simulink model "AFC_FFNN_trainlm_15_15_15_15_Apr_1_2020_M"  (R2021b)
settings: Solver=ode15s  StartTime=0.0  StopTime=30  MaxStep=0.01  RelTol=1e-3
libraries: neural x66
(part 3 of 3)

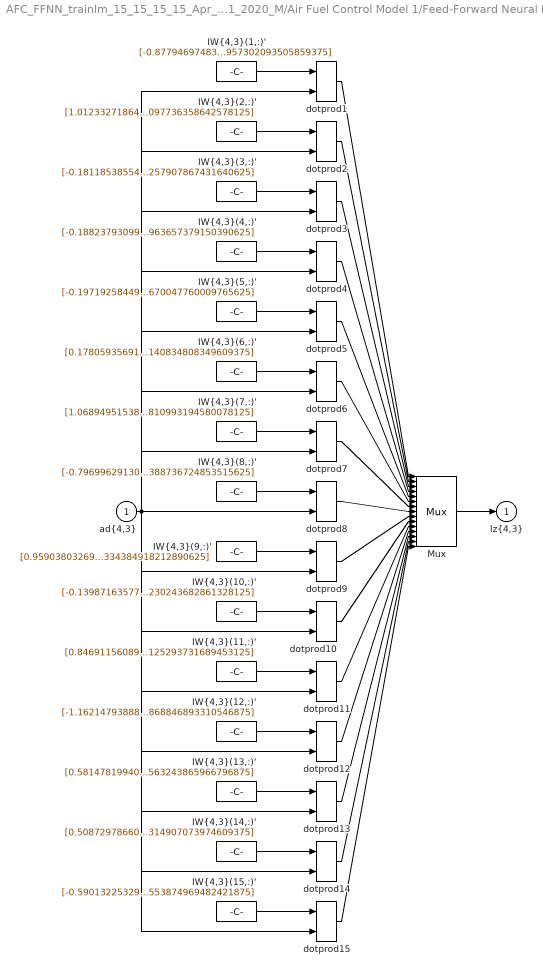
== system AFC_FFNN_trainlm_15_15_15_15_Apr_1_2020_M/Air Fuel Control Model 1/Feed-Forward Neural Network/Layer 4/LW{4,3} ==
  "ad{4,3}" : Inport  PortDimensions=15
      mask Display: e = 0.06;c1 = [120 230 180]/255;c2 = ([120 230 180]+0)/(256+128);c3 = ([120 230 180]+128)/(256+128);patch([0 1 1 0],[0 0 1 1],c1);patch([0 1 1 1-e 1-e 0+e],[0 0 1 1-e 0+e 0+e],c2);patch([0 0 1 1-e 0+e 0+e],[0 1 1 1-e 1-e 0+e],c3);plot([0 1 1 0 0],[0 0 1 1 0]);
  "IW{4,3}(1,:)'" : Constant  Value=[-0.87794697483855188568924177161534316837787628173828125;0.78511271343722122129094032061402685940265655517578125;0.50154215742376317965778298457735218107700347900390625;0.2817626613878057018069966943585313856601715087890625;-0.0447481608464237456956880123470909893512725830078125;-0.627329734092003210577104255207814276218414306640625;0.55694927688418560673966339891194365918636322021484375;-0.7464244490308360457930803022463805973529815673828125;0.54695272101903003036937889191904105246067047119140625;-0.30506713981724431494768623451818712055683135986328125;0.1330716598486472446172257377838832326233386993408203125;-0.36209291832798218280231594690121710300445556640625;0.1493922263287312812707341436180286109447479248046875;0.721901657154491172008192734210751950740814208984375;0.57616554688412902063276987973949871957302093505859375]
      mask Display: e = 0.06;c1 = [120 150 230]/255;c2 = ([120 150 230]+0)/383;c3 = ([120 150 230]+128)/383;patch([0 1 1 0],[0 0 1 1],c1);patch([0 1 1 1-e 1-e 0+e],[0 0 1 1-e 0+e 0+e],c2);patch([0 0 1 1-e 0+e 0+e],[0 1 1 1-e 1-e 0+e],c3);plot([0 1 1 0 0],[0 0 1 1 0]);disp('weights');
  "IW{4,3}(10,:)'" : Constant  Value=[-0.1398716357765525108991511160638765431940555572509765625;0.082048350523899193920129846446798183023929595947265625;0.0035940872365181979718185001360097885481081902980804443359375;0.61364753046270592573563362748245708644390106201171875;-0.1449570401924471507726366326096467673778533935546875;-0.621340313949121370029615718522109091281890869140625;-0.63152240904524414855103486843290738761425018310546875;0.18129030978633087212159580303705297410488128662109375;0.70918842566612350086785454550408758223056793212890625;0.444294267001949183537590215564705431461334228515625;0.3511170382244828136464320778031833469867706298828125;0.9678951234339694398300935063161887228488922119140625;-0.43500142397416130535248157684691250324249267578125;-0.292582299598873607493487725150771439075469970703125;-0.72720331825824502391952819380094297230243682861328125]
      mask Display: e = 0.06;c1 = [120 150 230]/255;c2 = ([120 150 230]+0)/383;c3 = ([120 150 230]+128)/383;patch([0 1 1 0],[0 0 1 1],c1);patch([0 1 1 1-e 1-e 0+e],[0 0 1 1-e 0+e 0+e],c2);patch([0 0 1 1-e 0+e 0+e],[0 1 1 1-e 1-e 0+e],c3);plot([0 1 1 0 0],[0 0 1 1 0]);disp('weights');
  "IW{4,3}(11,:)'" : Constant  Value=[0.8469115608906976344627537400810979306697845458984375;-0.311598694041631762985389286768622696399688720703125;-0.4555113193085655876046757839503698050975799560546875;0.2257560371225231232727992392028681933879852294921875;-0.1536297879854113812569949004682712256908416748046875;0.6246753040878669782642873542499728500843048095703125;-0.618342893403056592660504975356161594390869140625;0.87203667944872542694412231867318041622638702392578125;0.312036102352537036974666762034757994115352630615234375;0.53507958236281094599462448968552052974700927734375;1.0606246666988126126085489886463619768619537353515625;0.459631876268668915219706150310230441391468048095703125;0.87284799201372553767441786476410925388336181640625;0.3642501475629236207254280088818632066249847412109375;0.32478448388082625797323998995125293731689453125]
      mask Display: e = 0.06;c1 = [120 150 230]/255;c2 = ([120 150 230]+0)/383;c3 = ([120 150 230]+128)/383;patch([0 1 1 0],[0 0 1 1],c1);patch([0 1 1 1-e 1-e 0+e],[0 0 1 1-e 0+e 0+e],c2);patch([0 0 1 1-e 0+e 0+e],[0 1 1 1-e 1-e 0+e],c3);plot([0 1 1 0 0],[0 0 1 1 0]);disp('weights');
  "IW{4,3}(12,:)'" : Constant  Value=[-1.1621479388899036422344579477794468402862548828125;-0.88605701259143276882213058343040756881237030029296875;0.66235299370133871033061723210266791284084320068359375;-0.07077567879171035858387739381214487366378307342529296875;-0.27211799036489470182687000487931072711944580078125;0.72261696466571867514261384712881408631801605224609375;0.55103460441041873796308436794788576662540435791015625;0.183429125512546919996026417720713652670383453369140625;-0.344389971699303687469040369251160882413387298583984375;-0.91398906043296601620085084505262784659862518310546875;0.57553134575504871772722026435076259076595306396484375;-0.5461197652611726738314246176742017269134521484375;-0.708172309786351039662122275331057608127593994140625;0.3874597979113507673076810533530078828334808349609375;-0.9807440176240997953271971709909848868846893310546875]
      mask Display: e = 0.06;c1 = [120 150 230]/255;c2 = ([120 150 230]+0)/383;c3 = ([120 150 230]+128)/383;patch([0 1 1 0],[0 0 1 1],c1);patch([0 1 1 1-e 1-e 0+e],[0 0 1 1-e 0+e 0+e],c2);patch([0 0 1 1-e 0+e 0+e],[0 1 1 1-e 1-e 0+e],c3);plot([0 1 1 0 0],[0 0 1 1 0]);disp('weights');
  "IW{4,3}(13,:)'" : Constant  Value=[0.58147819940035194719030187116004526615142822265625;0.66671058191855803176650852037710137665271759033203125;0.82713190563479377370725842411047779023647308349609375;-0.7444983522659407437771506010903976857662200927734375;0.40638725377066275967763431253843009471893310546875;0.6613316222049554493622736117686145007610321044921875;0.80557784201437854232352719918708316981792449951171875;0.18716756979224313806042800933937542140483856201171875;0.65199814324099103490794959725462831556797027587890625;-0.851432769005782130733450685511343181133270263671875;-0.283226375762959836634991006576456129550933837890625;0.63658715279129207686992231174372136592864990234375;-0.4675533643194753619098946728627197444438934326171875;-0.3662417914291811182891933640348725020885467529296875;0.5858475047353255416027195678907446563243865966796875]
      mask Display: e = 0.06;c1 = [120 150 230]/255;c2 = ([120 150 230]+0)/383;c3 = ([120 150 230]+128)/383;patch([0 1 1 0],[0 0 1 1],c1);patch([0 1 1 1-e 1-e 0+e],[0 0 1 1-e 0+e 0+e],c2);patch([0 0 1 1-e 0+e 0+e],[0 1 1 1-e 1-e 0+e],c3);plot([0 1 1 0 0],[0 0 1 1 0]);disp('weights');
  "IW{4,3}(14,:)'" : Constant  Value=[0.5087297866062605589121403681929223239421844482421875;0.188991786837609809790450299260555766522884368896484375;0.62040033157972629407339582030544988811016082763671875;-1.3169260075057744874271747903549112379550933837890625;-0.29726006120487280526276663294993340969085693359375;0.58833087830961405817475906587787903845310211181640625;-0.647600995689554093104334242525510489940643310546875;-0.24550691338193553203694818876101635396480560302734375;-0.06475428417855148832682488091450068168342113494873046875;-0.8097839625485210302002769822138361632823944091796875;-0.69917278753788469902730184912797994911670684814453125;1.0912869846500914405851290212012827396392822265625;-0.5144129881700150175305452648899517953395843505859375;0.79022942493543701925062805457855574786663055419921875;2.26916884611590941034364732331596314907073974609375]
      mask Display: e = 0.06;c1 = [120 150 230]/255;c2 = ([120 150 230]+0)/383;c3 = ([120 150 230]+128)/383;patch([0 1 1 0],[0 0 1 1],c1);patch([0 1 1 1-e 1-e 0+e],[0 0 1 1-e 0+e 0+e],c2);patch([0 0 1 1-e 0+e 0+e],[0 1 1 1-e 1-e 0+e],c3);plot([0 1 1 0 0],[0 0 1 1 0]);disp('weights');
  "IW{4,3}(15,:)'" : Constant  Value=[-0.59013225329123086826399458004743792116641998291015625;0.68362536896318470969191594122094102203845977783203125;0.51268345737815590457131520452094264328479766845703125;0.73534210419389067769913026495487429201602935791015625;-0.722623441227063789682460992480628192424774169921875;0.4950531857779767452854002840467728674411773681640625;0.0039842636764119976344744600282865576446056365966796875;0.58761554450892272694062512528034858405590057373046875;-0.58080760878334014574164712030324153602123260498046875;-0.32518728515714634408340089066768996417522430419921875;0.8049732768928656856388670348678715527057647705078125;-0.34826732744436983413294228739687241613864898681640625;0.7186328066455740515294792203349061310291290283203125;-0.3212892271896301554789943111245520412921905517578125;0.334461971693696902274695048618013970553874969482421875]
      mask Display: e = 0.06;c1 = [120 150 230]/255;c2 = ([120 150 230]+0)/383;c3 = ([120 150 230]+128)/383;patch([0 1 1 0],[0 0 1 1],c1);patch([0 1 1 1-e 1-e 0+e],[0 0 1 1-e 0+e 0+e],c2);patch([0 0 1 1-e 0+e 0+e],[0 1 1 1-e 1-e 0+e],c3);plot([0 1 1 0 0],[0 0 1 1 0]);disp('weights');
  "IW{4,3}(2,:)'" : Constant  Value=[1.0123327186491437590376563093741424381732940673828125;1.098571239363774765251946519128978252410888671875;1.0135981388833539273974793104571290314197540283203125;0.190480505210553541228790663808467797935009002685546875;-0.61174606671621578612985103973187506198883056640625;0.001871022357728312213165366983957937918603420257568359375;-0.77443426081876098887590842423378489911556243896484375;0.8933686526028079555317162885330617427825927734375;-0.05576797680758034669867839738799375481903553009033203125;0.337953956266565713750793520375736989080905914306640625;-0.1422828298717915551652168915097718127071857452392578125;0.7575526069568947473698017347487621009349822998046875;-0.4194139141820738547750124780577607452869415283203125;0.66597243693851115864390521892346441745758056640625;-0.83251762673654561286440412004594691097736358642578125]
      mask Display: e = 0.06;c1 = [120 150 230]/255;c2 = ([120 150 230]+0)/383;c3 = ([120 150 230]+128)/383;patch([0 1 1 0],[0 0 1 1],c1);patch([0 1 1 1-e 1-e 0+e],[0 0 1 1-e 0+e 0+e],c2);patch([0 0 1 1-e 0+e 0+e],[0 1 1 1-e 1-e 0+e],c3);plot([0 1 1 0 0],[0 0 1 1 0]);disp('weights');
  "IW{4,3}(3,:)'" : Constant  Value=[-0.1811853855497163878762734157135128043591976165771484375;-0.5960881500003465394144086531014181673526763916015625;0.441979396271819202635100509723997674882411956787109375;0.7947734403244870460270021794713102281093597412109375;-0.1868516521181187162170544979744590818881988525390625;-1.0137783650240865807035106627154164016246795654296875;0.33786822212746570048835792476893402636051177978515625;0.40355475766253279257256281198351643979549407958984375;0.420947115571197294503491548312013037502765655517578125;-0.926163186954993111754674828262068331241607666015625;0.223759547769176114773159724791184999048709869384765625;0.8695239017841422946020202289219014346599578857421875;-0.4197462449481268453865823175874538719654083251953125;0.8011093081199256449309586969320662319660186767578125;0.018384635967900353481496722451993264257907867431640625]
      mask Display: e = 0.06;c1 = [120 150 230]/255;c2 = ([120 150 230]+0)/383;c3 = ([120 150 230]+128)/383;patch([0 1 1 0],[0 0 1 1],c1);patch([0 1 1 1-e 1-e 0+e],[0 0 1 1-e 0+e 0+e],c2);patch([0 0 1 1-e 0+e 0+e],[0 1 1 1-e 1-e 0+e],c3);plot([0 1 1 0 0],[0 0 1 1 0]);disp('weights');
  "IW{4,3}(4,:)'" : Constant  Value=[-0.1882379309967188996122189337256713770329952239990234375;0.89920767196481643512839809773140586912631988525390625;-0.7963876016425033288470558545668609440326690673828125;-0.00942815664871557955473146961367092444561421871185302734375;0.829359092604627701206254641874693334102630615234375;0.386189766269589729308364667303976602852344512939453125;0.56148647590458555800552176151541061699390411376953125;-0.7148532027965293078608510768390260636806488037109375;0.206937721753990666595512948333634994924068450927734375;0.265127551825350249448121076056850142776966094970703125;-0.288570537994503606427088016062043607234954833984375;0.55649333418204793844097366672940552234649658203125;-0.8044316294032711756045728179742582142353057861328125;0.5612939377825572062619130520033650100231170654296875;0.73878778787138055239580580746405757963657379150390625]
      mask Display: e = 0.06;c1 = [120 150 230]/255;c2 = ([120 150 230]+0)/383;c3 = ([120 150 230]+128)/383;patch([0 1 1 0],[0 0 1 1],c1);patch([0 1 1 1-e 1-e 0+e],[0 0 1 1-e 0+e 0+e],c2);patch([0 0 1 1-e 0+e 0+e],[0 1 1 1-e 1-e 0+e],c3);plot([0 1 1 0 0],[0 0 1 1 0]);disp('weights');
  "IW{4,3}(5,:)'" : Constant  Value=[-0.197192584497892564598942044540308415889739990234375;-0.5186706284037716496726488912827335298061370849609375;0.510598952565356256627637776546180248260498046875;-0.5671754650160829580585186704411171376705169677734375;0.6290541607610642405035150659386999905109405517578125;-0.593972205237285333367935891146771609783172607421875;0.56367557776157273252692903042770922183990478515625;-0.2391886933281599514344861745485104620456695556640625;0.2483531137671775024244880114565603435039520263671875;-0.4021721998758012173169618108659051358699798583984375;-0.8607509458168005611611306449049152433872222900390625;-0.6985358795817571131436807263526134192943572998046875;0.09485220801825988701239111833274364471435546875;-0.42931368309029682706068342668004333972930908203125;0.1919537785317848577193444725708104670047760009765625]
      mask Display: e = 0.06;c1 = [120 150 230]/255;c2 = ([120 150 230]+0)/383;c3 = ([120 150 230]+128)/383;patch([0 1 1 0],[0 0 1 1],c1);patch([0 1 1 1-e 1-e 0+e],[0 0 1 1-e 0+e 0+e],c2);patch([0 0 1 1-e 0+e 0+e],[0 1 1 1-e 1-e 0+e],c3);plot([0 1 1 0 0],[0 0 1 1 0]);disp('weights');
  "IW{4,3}(6,:)'" : Constant  Value=[0.1780593569155609345866508874678402207791805267333984375;0.51295577667334602001147914052125997841358184814453125;-0.2488674401089323584557178037357516586780548095703125;-0.52678522851250020320179601185373030602931976318359375;0.2838564984986617911744133380125276744365692138671875;0.7661743777528631227369260159321129322052001953125;-0.395950144348631460911036583638633601367473602294921875;0.66942143988391222819700487889349460601806640625;-0.70887282503045512260797522685606963932514190673828125;0.420234137501336479925129196999478153884410858154296875;-0.3134912186981633208660014133783988654613494873046875;-0.31435256189060167830717773540527559816837310791015625;0.244775657654162426268840135890059173107147216796875;0.55164477009675305652081078733317553997039794921875;-0.332656944910989016417346419984824024140834808349609375]
      mask Display: e = 0.06;c1 = [120 150 230]/255;c2 = ([120 150 230]+0)/383;c3 = ([120 150 230]+128)/383;patch([0 1 1 0],[0 0 1 1],c1);patch([0 1 1 1-e 1-e 0+e],[0 0 1 1-e 0+e 0+e],c2);patch([0 0 1 1-e 0+e 0+e],[0 1 1 1-e 1-e 0+e],c3);plot([0 1 1 0 0],[0 0 1 1 0]);disp('weights');
  "IW{4,3}(7,:)'" : Constant  Value=[1.0689495153859998044509893588838167488574981689453125;-0.48233115858616770754707658852566964924335479736328125;0.0623997962497397640202478896753746084868907928466796875;0.7931784702682118659566867790999822318553924560546875;-0.1412504172778643596330994114396162331104278564453125;0.354917548973855356830853224892052821815013885498046875;0.82917133329300707345055343466810882091522216796875;-0.01606084327905706043981837183309835381805896759033203125;-0.50281957762533469047383505312609486281871795654296875;-0.55237366074994465048320080313715152442455291748046875;-0.69503012315862633396790215556393377482891082763671875;0.5879995412831016121657512485398910939693450927734375;0.2442786986054261699763401338714174926280975341796875;-0.906706083575766541571283596567809581756591796875;-0.79723882076575158794895514802192337810993194580078125]
      mask Display: e = 0.06;c1 = [120 150 230]/255;c2 = ([120 150 230]+0)/383;c3 = ([120 150 230]+128)/383;patch([0 1 1 0],[0 0 1 1],c1);patch([0 1 1 1-e 1-e 0+e],[0 0 1 1-e 0+e 0+e],c2);patch([0 0 1 1-e 0+e 0+e],[0 1 1 1-e 1-e 0+e],c3);plot([0 1 1 0 0],[0 0 1 1 0]);disp('weights');
  "IW{4,3}(8,:)'" : Constant  Value=[-0.79699629130861981973765750808524899184703826904296875;0.81516845271742022216443501747562550008296966552734375;-0.10325580243793168466748255696074920706450939178466796875;-0.12629156005249997374306758501916192471981048583984375;0.001780542089853565101975618745200335979461669921875;-0.626000500890068867221316395443864166736602783203125;0.022190916577181425684006654819313553161919116973876953125;-0.161612416675443737457129600443295203149318695068359375;-0.278241324625298769301906531836721114814281463623046875;-0.5271108348563908752026918591582216322422027587890625;1.044387681269747236711964433197863399982452392578125;0.6362087423169793254373871604911983013153076171875;-0.3089480363396763795691413179156370460987091064453125;0.209791869896167992859403739203116856515407562255859375;1.9123701938083981222149532186449505388736724853515625]
      mask Display: e = 0.06;c1 = [120 150 230]/255;c2 = ([120 150 230]+0)/383;c3 = ([120 150 230]+128)/383;patch([0 1 1 0],[0 0 1 1],c1);patch([0 1 1 1-e 1-e 0+e],[0 0 1 1-e 0+e 0+e],c2);patch([0 0 1 1-e 0+e 0+e],[0 1 1 1-e 1-e 0+e],c3);plot([0 1 1 0 0],[0 0 1 1 0]);disp('weights');
  "IW{4,3}(9,:)'" : Constant  Value=[0.95903803269837906153583162449649535119533538818359375;0.1797639268302933801546572567531256936490535736083984375;0.47397786629673699376752438183757476508617401123046875;0.84812206479178875451196972790057770907878875732421875;-0.6216250145664379278542810425278730690479278564453125;1.0559711154374264996391730164759792387485504150390625;1.003550640057164766716368831112049520015716552734375;-0.16921524677973753814086421698448248207569122314453125;-0.388523293891599064142639008423429913818836212158203125;0.64295138099676096832268967773416079580783843994140625;-0.7218467335780027749336795750423334538936614990234375;0.755669871799011350077535098535008728504180908203125;-0.7771348063268403993930633077980019152164459228515625;-0.9635683972860367152435401294496841728687286376953125;0.0846822230062286573915031340220593847334384918212890625]
      mask Display: e = 0.06;c1 = [120 150 230]/255;c2 = ([120 150 230]+0)/383;c3 = ([120 150 230]+128)/383;patch([0 1 1 0],[0 0 1 1],c1);patch([0 1 1 1-e 1-e 0+e],[0 0 1 1-e 0+e 0+e],c2);patch([0 0 1 1-e 0+e 0+e],[0 1 1 1-e 1-e 0+e],c3);plot([0 1 1 0 0],[0 0 1 1 0]);disp('weights');
  Mux : Mux  Inputs=15
      mask Display: e = 0.06;c1 = [120 150 230]/255;c2 = ([120 150 230]+0)/383;c3 = ([120 150 230]+128)/383;patch([0 1 1 0],[0 0 1 1],c1);patch([0 1 1 1-e 1-e 0+e],[0 0 1 1-e 0+e 0+e],c2);patch([0 0 1 1-e 0+e 0+e],[0 1 1 1-e 1-e 0+e],c3);plot([0 1 1 0 0],[0 0 1 1 0]);disp('Mux');
  dotprod{1..15} (15 alike) : neural/Weight Functions/dotprod
  "lz{4,3}" : Outport
      mask Display: e = 0.06;c1 = [120 230 180]/255;c2 = ([120 230 180]+0)/(256+128);c3 = ([120 230 180]+128)/(256+128);patch([0 1 1 0],[0 0 1 1],c1);patch([0 1 1 1-e 1-e 0+e],[0 0 1 1-e 0+e 0+e],c2);patch([0 0 1 1-e 0+e 0+e],[0 1 1 1-e 1-e 0+e],c3);plot([0 1 1 0 0],[0 0 1 1 0]);
  wires:
  "IW{4,3}(1,:)'"/1 -> dotprod1/1
  "ad{4,3}"/1 -> dotprod1/2, dotprod2/2, dotprod3/2, dotprod4/2, dotprod5/2, dotprod6/2, dotprod7/2, dotprod8/2, dotprod9/2, dotprod10/2, dotprod11/2, dotprod12/2, dotprod13/2, dotprod14/2, dotprod15/2
  dotprod1/1 -> Mux/1
  "IW{4,3}(2,:)'"/1 -> dotprod2/1
  dotprod2/1 -> Mux/2
  "IW{4,3}(3,:)'"/1 -> dotprod3/1
  dotprod3/1 -> Mux/3
  "IW{4,3}(4,:)'"/1 -> dotprod4/1
  dotprod4/1 -> Mux/4
  "IW{4,3}(5,:)'"/1 -> dotprod5/1
  dotprod5/1 -> Mux/5
  "IW{4,3}(6,:)'"/1 -> dotprod6/1
  dotprod6/1 -> Mux/6
  "IW{4,3}(7,:)'"/1 -> dotprod7/1
  dotprod7/1 -> Mux/7
  "IW{4,3}(8,:)'"/1 -> dotprod8/1
  dotprod8/1 -> Mux/8
  "IW{4,3}(9,:)'"/1 -> dotprod9/1
  dotprod9/1 -> Mux/9
  "IW{4,3}(10,:)'"/1 -> dotprod10/1
  dotprod10/1 -> Mux/10
  "IW{4,3}(11,:)'"/1 -> dotprod11/1
  dotprod11/1 -> Mux/11
  "IW{4,3}(12,:)'"/1 -> dotprod12/1
  dotprod12/1 -> Mux/12
  "IW{4,3}(13,:)'"/1 -> dotprod13/1
  dotprod13/1 -> Mux/13
  "IW{4,3}(14,:)'"/1 -> dotprod14/1
  dotprod14/1 -> Mux/14
  "IW{4,3}(15,:)'"/1 -> dotprod15/1
  dotprod15/1 -> Mux/15
  Mux/1 -> "lz{4,3}"/1

== system AFC_FFNN_trainlm_15_15_15_15_Apr_1_2020_M/Air Fuel Control Model 1/Feed-Forward Neural Network/Layer 5/Delays 1 ==
  "p{5}" : Inport  PortDimensions=15
      mask Display: e = 0.06;c1 = [120 230 180]/255;c2 = ([120 230 180]+0)/(256+128);c3 = ([120 230 180]+128)/(256+128);patch([0 1 1 0],[0 0 1 1],c1);patch([0 1 1 1-e 1-e 0+e],[0 0 1 1-e 0+e 0+e],c2);patch([0 0 1 1-e 0+e 0+e],[0 1 1 1-e 1-e 0+e],c3);plot([0 1 1 0 0],[0 0 1 1 0]);
  mux : Mux  Inputs=1
      mask Display: e = 0.06;c1 = [120 150 230]/255;c2 = ([120 150 230]+0)/383;c3 = ([120 150 230]+128)/383;patch([0 1 1 0],[0 0 1 1],c1);patch([0 1 1 1-e 1-e 0+e],[0 0 1 1-e 0+e 0+e],c2);patch([0 0 1 1-e 0+e 0+e],[0 1 1 1-e 1-e 0+e],c3);plot([0 1 1 0 0],[0 0 1 1 0]);disp('Mux')
  "pd{5,4}" : Outport
      mask Display: e = 0.06;c1 = [120 230 180]/255;c2 = ([120 230 180]+0)/(256+128);c3 = ([120 230 180]+128)/(256+128);patch([0 1 1 0],[0 0 1 1],c1);patch([0 1 1 1-e 1-e 0+e],[0 0 1 1-e 0+e 0+e],c2);patch([0 0 1 1-e 0+e 0+e],[0 1 1 1-e 1-e 0+e],c3);plot([0 1 1 0 0],[0 0 1 1 0]);
  wires:
  "p{5}"/1 -> mux/1
  mux/1 -> "pd{5,4}"/1

== system AFC_FFNN_trainlm_15_15_15_15_Apr_1_2020_M/Air Fuel Control Model 1/Feed-Forward Neural Network/Layer 5/LW{5,4} ==
  "ad{5,4}" : Inport  PortDimensions=15
      mask Display: e = 0.06;c1 = [120 230 180]/255;c2 = ([120 230 180]+0)/(256+128);c3 = ([120 230 180]+128)/(256+128);patch([0 1 1 0],[0 0 1 1],c1);patch([0 1 1 1-e 1-e 0+e],[0 0 1 1-e 0+e 0+e],c2);patch([0 0 1 1-e 0+e 0+e],[0 1 1 1-e 1-e 0+e],c3);plot([0 1 1 0 0],[0 0 1 1 0]);
  "IW{5,4}(1,:)'" : Constant  Value=[0.19989144575989870045162888345657847821712493896484375;0.52004998107383826333460774549166671931743621826171875;-0.752803453565191293961333940387703478336334228515625;0.428612666235617612020547539941617287695407867431640625;0.585595362040919109603009928832761943340301513671875;-0.3562629890878257210573565316735766828060150146484375;0.5961351434564565732188157198834232985973358154296875;-0.74671233793534808054204177096835337579250335693359375;0.311648142554934948211808887208462692797183990478515625;-0.66544677705073718154693551696254871785640716552734375;0.6726563067034001530686282421811483800411224365234375;-0.65963526623929624737030508185853250324726104736328125;-0.377066482508966682729578678845427930355072021484375;0.1906180581610984192675317672183155082166194915771484375;0.1745649841584534234240067007704055868089199066162109375]
      mask Display: e = 0.06;c1 = [120 150 230]/255;c2 = ([120 150 230]+0)/383;c3 = ([120 150 230]+128)/383;patch([0 1 1 0],[0 0 1 1],c1);patch([0 1 1 1-e 1-e 0+e],[0 0 1 1-e 0+e 0+e],c2);patch([0 0 1 1-e 0+e 0+e],[0 1 1 1-e 1-e 0+e],c3);plot([0 1 1 0 0],[0 0 1 1 0]);disp('weights');
  Mux : Mux  Inputs=1
      mask Display: e = 0.06;c1 = [120 150 230]/255;c2 = ([120 150 230]+0)/383;c3 = ([120 150 230]+128)/383;patch([0 1 1 0],[0 0 1 1],c1);patch([0 1 1 1-e 1-e 0+e],[0 0 1 1-e 0+e 0+e],c2);patch([0 0 1 1-e 0+e 0+e],[0 1 1 1-e 1-e 0+e],c3);plot([0 1 1 0 0],[0 0 1 1 0]);disp('Mux');
  dotprod1 : neural/Weight Functions/dotprod
  "lz{5,4}" : Outport
      mask Display: e = 0.06;c1 = [120 230 180]/255;c2 = ([120 230 180]+0)/(256+128);c3 = ([120 230 180]+128)/(256+128);patch([0 1 1 0],[0 0 1 1],c1);patch([0 1 1 1-e 1-e 0+e],[0 0 1 1-e 0+e 0+e],c2);patch([0 0 1 1-e 0+e 0+e],[0 1 1 1-e 1-e 0+e],c3);plot([0 1 1 0 0],[0 0 1 1 0]);
  wires:
  "IW{5,4}(1,:)'"/1 -> dotprod1/1
  "ad{5,4}"/1 -> dotprod1/2
  dotprod1/1 -> Mux/1
  Mux/1 -> "lz{5,4}"/1
